simulink model "problem1sml"  (R2023a)
settings: Solver=VariableStepAuto  StartTime=0.0  StopTime=30  RelTol=1e-3
settings Model: Creator=USER  LastModifiedBy=USER

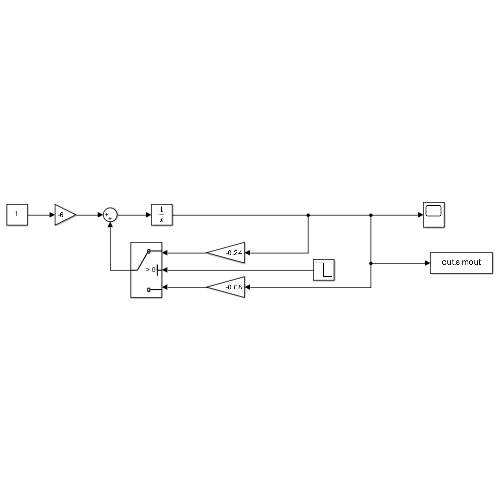
[thumbnail: Simulink's stored preview of the top-level diagram]
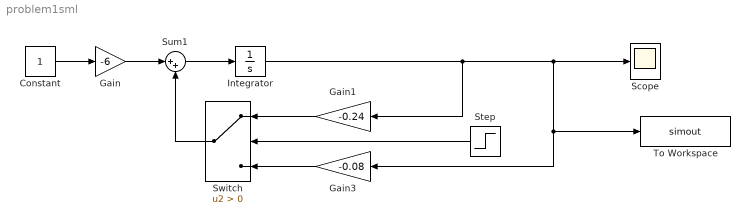
== system problem1sml ==
  Constant : Constant
  Gain : Gain  Gain=-6
  Gain1 : Gain  Gain=-0.24
  Gain3 : Gain  Gain=-0.08
  Integrator : Integrator  InitialCondition=-75
  Scope : Scope
  Step : Step  Before=1  After=0  SampleTime=0
  Sum1 : Sum  Inputs=|++
  Switch : Switch  Criteria=u2 > Threshold  SaturateOnIntegerOverflow=off  InputSameDT=off
  To Workspace : ToWorkspace  VariableName=simout  SaveFormat=Timeseries  SampleTime=-1
  wires:
  Sum1/1 -> Integrator/1
  Gain/1 -> Sum1/1
  Gain1/1 -> Switch/1
  Integrator/1 -> To Workspace/1, Gain3/1, Scope/1, Gain1/1
  Constant/1 -> Gain/1
  Step/1 -> Switch/2
  Gain3/1 -> Switch/3
  Switch/1 -> Sum1/2
